simulink model "top_model"  (R2024b)
settings: Solver=VariableStepAuto  StartTime=0.0  StopTime=90  RelTol=1e-3  EnableMultiTasking=on
values from neighbouring files (symbols this model uses):
  target = waypoints(idx, :)'    [waypointFollower - Copy.m]    (also in waypointFollower.m)
undefined symbols (not defined in the file or in its folder): controller, gray, vehicle, X, Y, Z
libraries: sm_lib x13, nesl_utility x6, simulink x5, slpidlib x2, robotmobilelib x1, deeplib x1, visionsinks x1
(part 2 of 2)

== matlab function top_model/###Recovered Stateflow Charts###/Visual Sensor Model_MATLAB Function_repaired_1 ==
  data: dx output; dy output; distance output; target_angle output; heading_error output; vehiclePose input; objectPos input; I output; ballRadius input; ballColor input
function [dx, dy, distance, target_angle, heading_error, I] = fakeCameraPOV(vehiclePose, objectPos, ballRadius, ballColor)
% Simulate a camera image from the vehicle's point of view, indicating if the target is in FOV.
% Inputs:
%   vehiclePose: [x_v; y_v; theta_v] - vehicle's world position (x_v, y_v) and heading (theta_v in radians)
%   objectPos: [x_o; y_o] - object's world position from figureEightPath
%   ballRadius: scalar - radius of the ball in world units (unused)
%   ballColor: 1×3 vector [R G B] - color of the ball
% Output:
%   I: H×W×3 uint8 image for Simulink Video Viewer (target color if in FOV, black if not)

% Image dimensions
H = 224; W = 224;
I = zeros(H, W, 3, 'uint8'); % Initialize black image

% Camera parameters
max_distance = 20; % Maximum viewable distance (matches world size)
fov = deg2rad(120); % Field of view (120 degrees)

% Extract inputs
x_v = vehiclePose(1); y_v = vehiclePose(2); theta_v = vehiclePose(3);
x_o = objectPos(1); y_o = objectPos(2);

% Compute direct distance in world frame
dx = x_o - x_v;
dy = y_o - y_v;
% dx = x_v - x_o;
% dy = y_v - y_o;
distance = sqrt(dx^2 + dy^2);

% Compute angle to target in world frame
target_angle = atan2(dy, dx); % Angle of target relative to positive x-axis

% Compute heading error (difference between robot heading and target angle)
heading_error = target_angle - theta_v;
heading_error = mod(heading_error + pi, 2*pi) - pi; % Normalize to [-pi, pi]

% Check if object is within range and FOV
if distance <= max_distance && abs(heading_error) <= fov/2
    % Target is in FOV: set image to target color
    I(:,:,1) = ballColor(1); % Red channel
    I(:,:,2) = ballColor(2); % Green channel
    I(:,:,3) = ballColor(3); % Blue channel
else
    % Target not in FOV: leave image black
    I = I; % Already black
end

end

== matlab function top_model/Waypoint Follower /MATLAB Function ==
  data: state input; target output; waypoints input; idxIn input; idxOut output
function [target, idxOut] = followWaypoints(state, waypoints, idxIn)
% state = [x; y; theta]
% waypoints = Nx2 array
% idxIn = current waypoint index
% target = [xTarget; yTarget]
% idxOut = updated waypoint index

threshold = 0.5;  % distance threshold (m)

% Current robot position
x = state(1);
y = state(2);

% Current waypoint target
target = waypoints(idxIn, :)';

% Check distance to waypoint
distance = norm([x; y] - target);

% If close to waypoint, move to next
if distance < threshold
    idxOut = mod(idxIn, size(waypoints, 1)) + 1; % wrap to start if needed
    target = waypoints(idxOut, :)';
else
    idxOut = idxIn;
end
end

== matlab function top_model/Visual Sensor Model/MATLAB Function1 ==
  data: scores input; labelName output; action output
function [labelName, action] = getLabel(scores)
    % Load class names (these must match your training set)
    classNames = ["Tomato___Bacterial_spot", ...
                  "Tomato___Early_blight", ...
                  "Tomato___Leaf_Mold", ...
                  "Tomato___healthy"];

    % Get the predicted class index
    [~, idx] = max(scores);
    labelName = classNames(idx);

    % Determine action based on class
    if contains(labelName, ["Bacterial", "blight", "Mold", "Virus", "Spider"])
        action = "Treat";
    elseif contains(labelName, "healthy")
        action = "No Action"; %or 'healthy'  , etc.
    else
        action = "Unknown";
    end
end
